simulink model "three"  (R2020b)
settings: Solver=FixedStepDiscrete  StartTime=0.0  StopTime=10  RelTol=1e-3
PreLoadFcn:
  | rad=2*pi
settings Model: Creator=USER  LastModifiedBy=USER

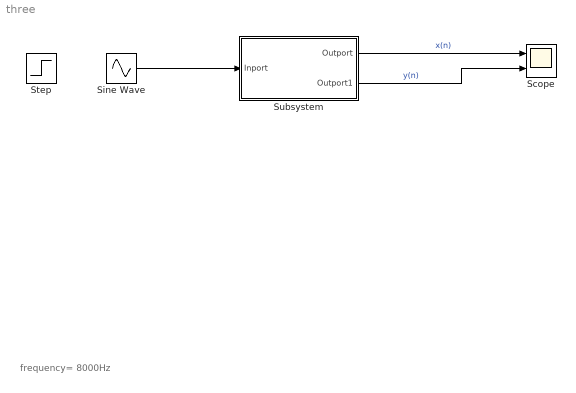
== system three ==
  note: frequency= 8000Hz
  Scope : Scope  NumInputPorts=2
  Sine Wave : Sin  Frequency=8000*rad  SampleTime=0
  Step : Step  SampleTime=0
  Subsystem : Subsystem
  wires:
  Subsystem/1(Outport) -> Scope/1  "x(n)"
  Subsystem/2(Outport1) -> Scope/2  "y(n)"
  Sine Wave/1 -> Subsystem/1(Inport)

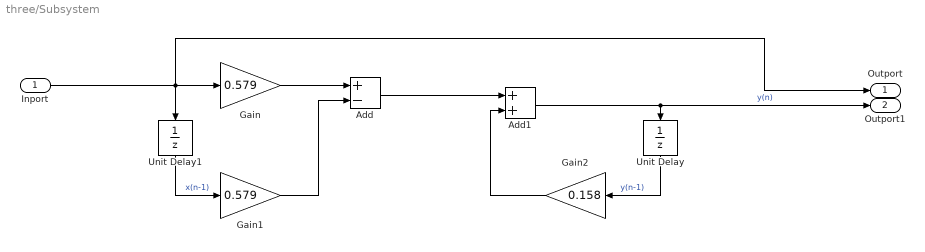
== system three/Subsystem ==
  Inport : Inport
  Add : Sum  Inputs=+-
  Add1 : Sum
  Gain : Gain  Gain=0.579
  Gain1 : Gain  Gain=0.579
  Gain2 : Gain  Gain=0.158
  Unit Delay : UnitDelay  SampleTime=-1  HasFrameUpgradeWarning=on
  Unit Delay1 : UnitDelay  SampleTime=-1  HasFrameUpgradeWarning=on
  Outport : Outport
  Outport1 : Outport  Port=2
  wires:
  Inport/1 -> Outport/1, Unit Delay1/1, Gain/1
  Add1/1 -> Outport1/1, Unit Delay/1  "y(n)"
  Add/1 -> Add1/1
  Gain1/1 -> Add/2
  Unit Delay1/1 -> Gain1/1  "x(n-1)"
  Unit Delay/1 -> Gain2/1  "y(n-1)"
  Gain/1 -> Add/1
  Gain2/1 -> Add1/2
